simulink model "CH13_3B"  (Simulink 9.2)
settings: Solver=ode45  StartTime=0.0  StopTime=5  RelTol=1e-3  EnableMultiTasking=on
libraries: dsparch4 x3, commsynccomp2 x1
settings Model: Creator=sw  LastModifiedBy=곽준영
settings DebuggingCC: SolverPrmCheckMsg=warning  StateNameClashWarn=none

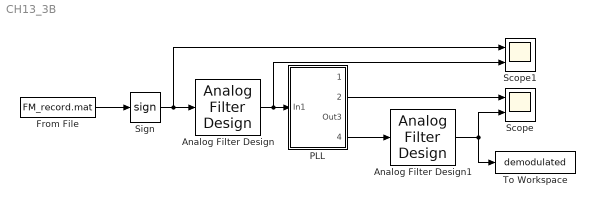
== system CH13_3B ==
  Analog Filter Design : dsparch4/Analog Filter Design  method=Butterworth  filttype=Bandpass  N=8  Wlo=2*pi*17.59461e3-2*pi*1e3  Whi=2*pi*17.59461e3+2*pi*1e3  Rp=2  Rs=40
  Analog Filter Design1 : dsparch4/Analog Filter Design  method=Butterworth  filttype=Lowpass  N=8  Wlo=4e3*2*pi  Whi=2.5e3*2*pi  Rp=2  Rs=40
  From File : FromFile  FileName=FM_record.mat
  PLL : Subsystem
  Scope : Scope  NumInputPorts=2
  Scope1 : Scope  NumInputPorts=2
  Sign : Signum
  To Workspace : ToWorkspace  VariableName=demodulated  SampleTime=1/(8192/3)
  wires:
  PLL/2(PD out) -> Scope/1
  PLL/4(VCO in) -> Analog Filter Design1/1
  Analog Filter Design1/1 -> Scope/2, To Workspace/1
  From File/1 -> Sign/1
  Analog Filter Design/1 -> Scope1/2, PLL/1(In1)
  Sign/1 -> Scope1/1, Analog Filter Design/1

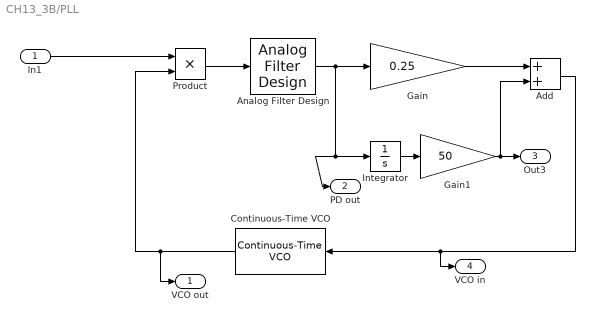
== system CH13_3B/PLL ==
  In1 : Inport
  Add : Sum
  Analog Filter Design : dsparch4/Analog Filter Design  method=Chebyshev II  filttype=Lowpass  N=32  Wlo=2*pi*4e3  Whi=80  Rp=2  Rs=40
  Continuous-Time VCO : commsynccomp2/Continuous-Time VCO  Ac=1  Fc=17.59461e3  Kc=1000  Ph=0
      settings: SourceProductName=Communications Toolbox  SourceProductBaseCode=CM
  Gain : Gain  Gain=0.25
  Gain1 : Gain  Gain=50
  Integrator : Integrator
  Product : Product  RndMeth=Zero
  VCO out : Outport
  PD out : Outport  Port=2
  Out3 : Outport  Port=3
  VCO in : Outport  Port=4
  wires:
  Product/1 -> Analog Filter Design/1
  Analog Filter Design/1 -> Gain/1, PD out/1, Integrator/1
  Gain/1 -> Add/1
  Integrator/1 -> Gain1/1
  Gain1/1 -> Add/2, Out3/1
  Add/1 -> Continuous-Time VCO/1, VCO in/1
  Continuous-Time VCO/1 -> VCO out/1, Product/2
  In1/1 -> Product/1
